simulink model "VSM_specComp_DC_22a"  (R2022a)
settings: Solver=ode3  StartTime=0.0  StopTime=4  FixedStep=HWSampleTime  RelTol=1e-3
PostLoadFcn:
  | EXEC_MODE=ExecutionMode.SIMULATION;
  | %Sim_TP33_VSM_HSS_init
InitFcn:
  | %EXEC_MODE=ExecutionMode.SIMULATION;
  | %Sim_TP33_VSM_HSS_init
StopFcn:
  | %sim2struct
undefined symbols (not defined in the file): ControlSampleTime, DiscIntNeverNeededParam, fault_dur, Grid, HWSampleTime, Ion, LCL, Lithium, Manage, Param, SM, t_fault, V_DC, VSMCTRL
libraries: FriedrichLibrary x76, simulink x32, TriphaseHardwaremodule x24, spsThreePhaseSeriesRLCBranchLib x8, spsThreePhaseVIMeasurementLib x8, spsThreePhaseBreakerLib x8, spsGroundLib x4, spsUniversalBridgeLib x4, spsVoltageMeasurementLib x4, spsEdgeDetectorLib x4, spsMeanLib x4, simulink_extras x4
(part 2 of 10)

== system VSM_specComp_DC_22a/VSM_1/VSM1/MeasInv1 ==
  SimOut : Inport
  Bus Selector1 : BusSelector  OutputSignals=meas_u_dc,meas_u_cap,meas_u_out,meas_i_inverter,meas_i_out,connection_state,enabled
  Meas_Inv1 : Scope  NumInputPorts=7
  To Workspace1 : ToWorkspace  VariableName=MeasAC_Ucap  SampleTime=-1
  To Workspace2 : ToWorkspace  VariableName=MeasAC_Uout  SampleTime=-1
  To Workspace3 : ToWorkspace  VariableName=MeasAC_Iinv  SampleTime=-1
  To Workspace4 : ToWorkspace  VariableName=MeasAC_Iout  SampleTime=-1
  To Workspace7 : ToWorkspace  VariableName=MeasAC_Udc  SampleTime=-1
  wires:
  Bus Selector1/7 -> Meas_Inv1/7  "<enabled>"
  Bus Selector1/6 -> Meas_Inv1/6  "<connection_state>"
  Bus Selector1/5 -> To Workspace4/1, Meas_Inv1/5  "<meas_i_out>"
  Bus Selector1/4 -> To Workspace3/1, Meas_Inv1/4  "<meas_i_inverter>"
  Bus Selector1/3 -> To Workspace2/1, Meas_Inv1/3  "<meas_u_out>"
  Bus Selector1/2 -> To Workspace1/1, Meas_Inv1/2  "<meas_u_cap>"
  Bus Selector1/1 -> To Workspace7/1, Meas_Inv1/1  "<meas_u_dc>"
  SimOut/1 -> Bus Selector1/1

== system VSM_specComp_DC_22a/VSM_1/VSM1/VSM ==
  cmd : Inport
  meas : Inport  Port=2
  BUS_GENERATION : Subsystem
  CONTROL : Subsystem
  MANAGEMENT : Subsystem  mask(VSMCC Management){Mgn=Ctrl.Mgn}
      mask prompts: Mgn "Mgn Parameters"
      mask help:
      | Mgn(.PQSpRateUp, .PQSpRateDown, PQSpMax, .PQSpMin)
      |
      | Parameter nicht auf der Maske:
      | ControlSampleTime
  Meas : Subsystem  mask(Messeinrichtung für VSM mit CC){PU=pu, PLL=Ctrl.PLL}
      mask prompts: PU "PU System"; PLL "PLL Parameters"
      mask help:
      | PU System(.Vb, .Ib)
      |
      | PLL Parameter (.kp, .ki)
      |
      | Parameter nicht auf der Maske:
      | NrChannels
      | ControlSampleTime
  ctrl : Outport  VectorParamsAs1DForOutWhenUnconnected=off  LockScale=on
  feedback : Outport  Port=2  VectorParamsAs1DForOutWhenUnconnected=off
  diag : Outport  Port=3  VectorParamsAs1DForOutWhenUnconnected=off
  wires:
  meas/1 -> Meas/1(MEASIN)
  cmd/1 -> MANAGEMENT/1(CMD)
  CONTROL/1(CONTROL) -> Meas/2("CONTROL "), BUS_GENERATION/2(CONTROL)
  BUS_GENERATION/1(ctrl) -> ctrl/1
  BUS_GENERATION/2(feedback) -> feedback/1
  CONTROL/2(diagCtrl) -> diag/1
  MANAGEMENT/1(MANAGE) -> CONTROL/1(MANAGE), BUS_GENERATION/1(MANAGE)
  Meas/1(MEAS) -> CONTROL/2(MEAS), MANAGEMENT/2(MEAS)

== system VSM_specComp_DC_22a/VSM_1/VSM1/command_center ==
  note: State Machine for TP <-> WP SIM
      |
      | State Index:
      | 0: Error
      | 1: Stop
      | 2: Ready (Precharge, Connected + Enable DC)
      | 3: Connect AC
      | 4: Enable AC
  Feed_AC : Inport
  Feed_DC : Inport  Port=2
  Bus Assignment : BusAssignment  AssignedSignals=Manage.connect,Manage.enable,Param.VSM.sp_PQ,Param.VSM.sp_E
  Bus Selector2 : BusSelector  OutputSignals=connect,enable
  Bus Creator1 : BusCreator  Inputs=2
  Constant2 : Constant  Value=1.01
  Display1 : Display
  Display2 : Display
  Display5 : Display
  Error ACK : Subsystem
      settings: OpenFcn=|
      | switch get_param([gcb '/Toggle'],'Value')
      |     case '1'
      |         set_param([gcb '/Toggle'],'Value', '0');
      |         set_param(gcb,'BackgroundColor','[0.8500    0.3250    0.0980]');
      |     case '0'
      |         set_param([gcb '/Toggle'],'Value', '1');
      |         set_param(gcb,'BackgroundColor','[0.4660    0.6740    0.1880]');
      | end
      mask Display: port_label('output',1,'')
  Rate Transition3 : RateTransition  Integrity=off  OutPortSampleTime=ControlSampleTime
  Shortcut1 : Subsystem  mask{path=./ControlLibrary/FriedrichLibrary.slx}
      settings: OpenFcn=findsimscopes
      mask Display: disp('Open Scopes...')
  Step3 : Step  Time=5.0+100  Before=[0.5 0]  After=[0.1 0]  SampleTime=0
  Step4 : Step  Time=0  SampleTime=0
  Subsystem : Subsystem
  cmd_VSM : Subsystem  AncestorBlock=ControLibrary/cmd_VSM template
  cmd_tp : Outport  VectorParamsAs1DForOutWhenUnconnected=off
  cmd_ac : Outport  Port=2  VectorParamsAs1DForOutWhenUnconnected=off
  wires:
  Rate Transition3/1 -> cmd_ac/1
  cmd_VSM/1(cmd_ac) -> Bus Assignment/1
  Bus Assignment/1 -> Rate Transition3/1
  Error ACK/1(Out) -> Bus Creator1/1  "error_ack"
  Bus Creator1/1 -> cmd_tp/1
  Subsystem/1(precharge) -> Bus Creator1/2, Display5/1
  Feed_AC/1 -> Subsystem/1(In1)
  Feed_DC/1 -> Subsystem/2(In2)
  Subsystem/2(cmd_ac) -> Bus Selector2/1
  Step4/1 -> Subsystem/Enable
  Step3/1 -> Bus Assignment/4
  Constant2/1 -> Bus Assignment/5
  Bus Selector2/1 -> Display1/1, Bus Assignment/2  "<connect>"
  Bus Selector2/2 -> Display2/1, Bus Assignment/3  "<enable>"

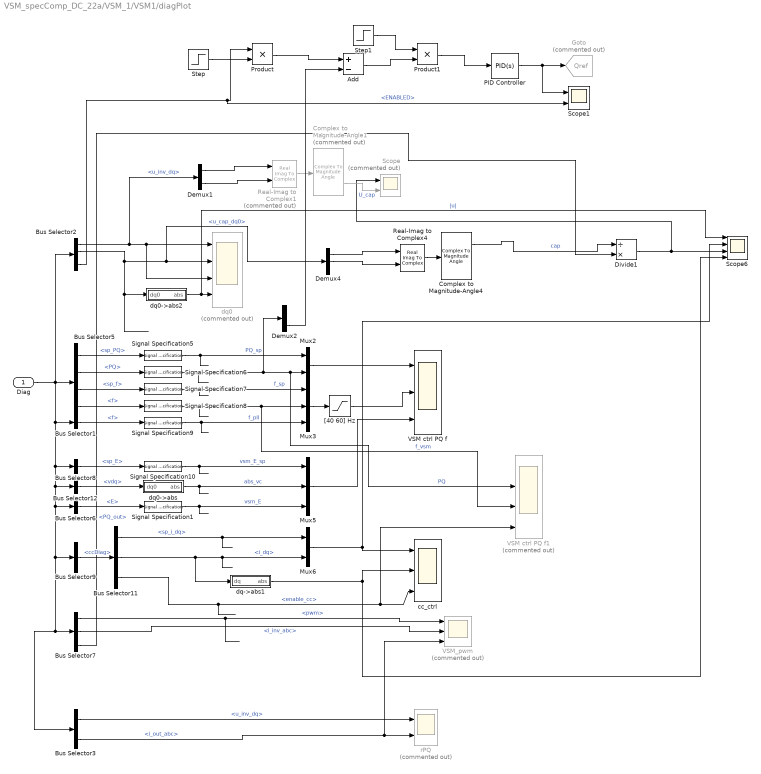
== system VSM_specComp_DC_22a/VSM_1/VSM1/diagPlot ==
  Diag : Inport
  Add : Sum  Inputs=+-
  Bus Selector1 : BusSelector  OutputSignals=measDiag.PLL.f
  Bus Selector11 : BusSelector  OutputSignals=sp_i_dq,i_dq,enable_cc
  Bus Selector12 : BusSelector  OutputSignals=measDiag.PLL.vdq
  Bus Selector2 : BusSelector  OutputSignals=u_inv_dq,measDiag.u_cap.u_cap_dq0,measDiag.u_cap.u_cap_abc,manage.ENABLED
  Bus Selector3 : BusSelector  OutputSignals=u_inv_dq,measDiag.i_out.i_out_abc
  Bus Selector5 : BusSelector  OutputSignals=manage.sp_VSM.sp_PQ,measDiag.PQ,manage.sp_VSM.sp_f,vsmDiag.f
  Bus Selector6 : BusSelector  OutputSignals=vsmDiag.E
  Bus Selector7 : BusSelector  OutputSignals=pwmDiag.pwm,measDiag.i_inv.i_inv_abc,measDiag.PQ_out
  Bus Selector8 : BusSelector  OutputSignals=vsmDiag.sp_VSM.sp_E
  Bus Selector9 : BusSelector  OutputSignals=ccDiag
  Complex to Magnitude-Angle1 : ComplexToMagnitudeAngle  Commented=on
  Complex to Magnitude-Angle4 : ComplexToMagnitudeAngle
  Demux1 : Demux  Outputs=2
  Demux2 : Demux  Outputs=2
  Demux4 : Demux  Outputs=3
  Divide1 : Product  Inputs=/*
  Goto : Goto  Commented=on  GotoTag=Qref  TagVisibility=global
  Mux2 : Mux  Inputs=2
  Mux3 : Mux  Inputs=3
  Mux5 : Mux  Inputs=3
  Mux6 : Mux  Inputs=2
  PID Controller : slpidlib/PID Controller  Controller=PID  Form=Parallel  TimeDomain=Continuous-time  UseExternalTs=off  SampleTime=-1  IntegratorMethod=Forward Euler  FilterMethod=Forward Euler  ControllerParametersSource=internal  P=0.1  I=1  UseKiTs=off  D=0  N=100  UseFilter=on  TunerSelectOption=Transfer Function Based (PID Tuner App)  InitialConditionSource=internal  InitialConditionForIntegrator=1.085  InitialConditionForFilter=0  DifferentiatorICPrevScaledInput=0  ExternalReset=none  TrackingMode=off  Kt=1  LimitOutput=off  SatLimitsSource=internal  UpperSaturationLimit=inf  LowerSaturationLimit=-inf  LinearizeAsGain=on  AntiWindupMode=none  Kb=1  POutMin=[]  POutMax=[]  IOutMin=[]  IOutMax=[]  DOutMin=[]  DOutMax=[]  NOutMin=[]  NOutMax=[]  SumOutMin=[]  SumOutMax=[]  SaturationOutMin=[]  SaturationOutMax=[]  PParamMin=[]  PParamMax=[]  IParamMin=[]  IParamMax=[]  DParamMin=[]  DParamMax=[]  NParamMin=[]  NParamMax=[]  KbParamMin=[]  KbParamMax=[]  KtParamMin=[]  KtParamMax=[]  KbOutMin=[]  KbOutMax=[]  KtOutMin=[]  KtOutMax=[]  IntegratorOutMin=[]  IntegratorOutMax=[]  FilterOutMin=[]  FilterOutMax=[]  SumI1OutMin=[]  SumI1OutMax=[]  SumI2OutMin=[]  SumI2OutMax=[]  SumI3OutMin=[]  SumI3OutMax=[]  SumI4OutMin=[]  SumI4OutMax=[]  SumDOutMin=[]  SumDOutMax=[]  DifferentiatorOutMin=[]  DifferentiatorOutMax=[]  FilterDiffOutCoefMin=[]  FilterDiffOutCoefMax=[]  ReciprocalOutMin=[]  ReciprocalOutMax=[]  SumDenOutMin=[]  SumDenOutMax=[]  SumNumOutMin=[]  SumNumOutMax=[]  DivideOutMin=[]  DivideOutMax=[]  UdiffTsProdOutMin=[]  UdiffTsProdOutMax=[]  NTsProdOutMin=[]  NTsProdOutMax=[]  UintegralTsProdOutMin=[]  UintegralTsProdOutMax=[]  UngainTsProdOutMin=[]  UngainTsProdOutMax=[]  IntegratorContinuousStateAttributes=''  IntegratorStateMustResolveToSignalObject=off  IntegratorRTWStateStorageClass=Auto  FilterContinuousStateAttributes=''  FilterStateMustResolveToSignalObject=off  FilterRTWStateStorageClass=Auto  ParallelPVariant=InternalParameters  IdealPVariant=Disabled  IVariant=InternalParameters  DVariant=InternalParameters  IntegratorVariant=Continuous  SatVariant=Disabled  AWVariant=Passthrough  PCopyVariant=Disabled  TRVariant=Disabled  FdbkBlocksVariant=Forward  IdealPFdbkVariant=Disabled  SatFdbkVariant=Disabled  DerivativeFilterVariant=ContFilter  NVariant=InternalParameters  NCopyVariant=Disabled  FilterICVariant=InternalICsFilter  IntegratorICVariant=InternalICs  ExternalResetVariant=Disabled  TRSumVariant=Passthrough  SumFdbkVariant=Disabled  SumVariant=Sum_PID  TsampFilterVariant=InternalTs  TsampNgainVariant=Passthrough  TsampIntegralVariant=Disabled_SignalSpec  ExternalSaturationOutDataTypeStr=Inherit: Same as second input
  Product : Product
  Product1 : Product
  Real-Imag to Complex1 : RealImagToComplex  Commented=on
  Real-Imag to Complex4 : RealImagToComplex
  Scope : Scope  Commented=on  NumInputPorts=2
  Scope1 : Scope  NumInputPorts=2
  Scope6 : Scope  NumInputPorts=4
  Signal Specification{1,5..10} (7 alike) : SignalSpecification
  Step : Step  Time=6+10  Before=0.1  After=0.5  SampleTime=0
  Step1 : Step  Time=6+10  SampleTime=0
  VSM ctrl PQ f : Scope  NumInputPorts=3
  VSM ctrl PQ f1 : Scope  Commented=on  NumInputPorts=4
  VSM_pwm : Scope  Commented=on  NumInputPorts=3
  "[40 60] Hz" : Saturate  UpperLimit=60  LowerLimit=40
  cc_ctrl : Scope  NumInputPorts=3
  dq->abs1 : Subsystem
  dq0 : Scope  Commented=on  NumInputPorts=4
  dq0->abs : Subsystem
  dq0->abs2 : Subsystem
  rPQ : Scope  Commented=on  NumInputPorts=2
  wires:
  Diag/1 -> Bus Selector2/1, Bus Selector6/1, Bus Selector7/1, Bus Selector3/1, Bus Selector9/1, Bus Selector12/1, Bus Selector8/1, Bus Selector1/1, Bus Selector5/1
  Bus Selector7/1 -> VSM_pwm/1  "<pwm>"
  Mux5/1 -> VSM ctrl PQ f/3
  dq0->abs/1(abs) -> Mux5/2  "abs_vc"
  Bus Selector8/1 -> Signal Specification10/1  "<sp_E>"
  Bus Selector11/1 -> Mux6/1  "<sp_i_dq>"
  Bus Selector9/1 -> Bus Selector11/1  "<ccDiag>"
  Bus Selector12/1 -> dq0->abs/1(dq0)  "<vdq>"
  Bus Selector11/3 -> VSM ctrl PQ f1/4, cc_ctrl/3  "<enable_cc>"
  Mux6/1 -> Scope6/2, cc_ctrl/1
  Bus Selector5/1 -> Signal Specification5/1  "<sp_PQ>"
  Bus Selector5/2 -> Signal Specification6/1  "<PQ>"
  Bus Selector5/3 -> Signal Specification7/1  "<sp_f>"
  Bus Selector5/4 -> Signal Specification8/1  "<f>"
  Signal Specification5/1 -> Mux2/1  "PQ_sp"
  Signal Specification7/1 -> Mux3/1  "f_sp"
  Signal Specification8/1 -> VSM ctrl PQ f1/3, Mux3/2  "f_vsm"
  Mux2/1 -> VSM ctrl PQ f/1
  Mux3/1 -> "[40 60] Hz"/1
  Bus Selector1/1 -> Signal Specification9/1  "<f>"
  Signal Specification9/1 -> Mux3/3  "f_pll"
  Signal Specification10/1 -> Mux5/1  "vsm_E_sp"
  Bus Selector11/2 -> dq->abs1/1(dq), Mux6/2  "<i_dq>"
  dq->abs1/1(abs) -> cc_ctrl/2, Scope6/4
  Bus Selector6/1 -> Signal Specification1/1  "<E>"
  Signal Specification1/1 -> Mux5/3  "vsm_E"
  "[40 60] Hz"/1 -> VSM ctrl PQ f/2
  dq0->abs2/1(abs) -> Scope6/1, dq0/4  "|u|"
  Bus Selector3/2 -> VSM_pwm/3, rPQ/2  "<i_out_abc>"
  Bus Selector3/1 -> rPQ/1  "<u_inv_dq>"
  Bus Selector7/2 -> VSM_pwm/2  "<i_inv_abc>"
  Bus Selector2/2 -> dq0->abs2/1(dq0), Demux4/1, dq0/2  "<u_cap_dq0>"
  Real-Imag to Complex4/1 -> Complex to Magnitude-Angle4/1
  Demux4/1 -> Real-Imag to Complex4/1
  Demux4/2 -> Real-Imag to Complex4/2
  Complex to Magnitude-Angle4/1 -> Divide1/1  "cap"
  Signal Specification6/1 -> Demux2/1, VSM ctrl PQ f1/2, Mux2/2  "PQ"
  Bus Selector7/3 -> Divide1/2  "<PQ_out>"
  Divide1/1 -> Scope/1, Scope6/3
  Demux1/2 -> Real-Imag to Complex1/2
  Demux1/1 -> Real-Imag to Complex1/1
  Real-Imag to Complex1/1 -> Complex to Magnitude-Angle1/1
  Complex to Magnitude-Angle1/2 -> Scope/2  "U_cap"
  Bus Selector2/1 -> Demux1/1, dq0/3, dq0/1  "<u_inv_dq>"
  Demux2/2 -> Add/2
  PID Controller/1 -> Scope1/1, Goto/1
  Step/1 -> Product/2
  Product/1 -> Add/1
  Bus Selector2/4 -> Scope1/2, Product/1  "<ENABLED>"
  Add/1 -> Product1/2
  Product1/1 -> PID Controller/1
  Step1/1 -> Product1/1

== system VSM_specComp_DC_22a/VSM_2/VSM1/MeasInv1 ==
  SimOut : Inport
  Bus Selector1 : BusSelector  OutputSignals=meas_u_dc,meas_u_cap,meas_u_out,meas_i_inverter,meas_i_out,connection_state,enabled
  Meas_Inv1 : Scope  NumInputPorts=7
  To Workspace1 : ToWorkspace  VariableName=MeasAC_Ucap  SampleTime=-1
  To Workspace2 : ToWorkspace  VariableName=MeasAC_Uout  SampleTime=-1
  To Workspace3 : ToWorkspace  VariableName=MeasAC_Iinv  SampleTime=-1
  To Workspace4 : ToWorkspace  VariableName=MeasAC_Iout  SampleTime=-1
  To Workspace7 : ToWorkspace  VariableName=MeasAC_Udc  SampleTime=-1
  wires:
  Bus Selector1/7 -> Meas_Inv1/7  "<enabled>"
  Bus Selector1/6 -> Meas_Inv1/6  "<connection_state>"
  Bus Selector1/5 -> To Workspace4/1, Meas_Inv1/5  "<meas_i_out>"
  Bus Selector1/4 -> To Workspace3/1, Meas_Inv1/4  "<meas_i_inverter>"
  Bus Selector1/3 -> To Workspace2/1, Meas_Inv1/3  "<meas_u_out>"
  Bus Selector1/2 -> To Workspace1/1, Meas_Inv1/2  "<meas_u_cap>"
  Bus Selector1/1 -> To Workspace7/1, Meas_Inv1/1  "<meas_u_dc>"
  SimOut/1 -> Bus Selector1/1

== system VSM_specComp_DC_22a/VSM_2/VSM1/VSM ==
  cmd : Inport
  meas : Inport  Port=2
  BUS_GENERATION : Subsystem
  CONTROL : Subsystem
  MANAGEMENT : Subsystem  mask(VSMCC Management){Mgn=Ctrl.Mgn}
      mask prompts: Mgn "Mgn Parameters"
      mask help:
      | Mgn(.PQSpRateUp, .PQSpRateDown, PQSpMax, .PQSpMin)
      |
      | Parameter nicht auf der Maske:
      | ControlSampleTime
  Meas : Subsystem  mask(Messeinrichtung für VSM mit CC){PU=pu, PLL=Ctrl.PLL}
      mask prompts: PU "PU System"; PLL "PLL Parameters"
      mask help:
      | PU System(.Vb, .Ib)
      |
      | PLL Parameter (.kp, .ki)
      |
      | Parameter nicht auf der Maske:
      | NrChannels
      | ControlSampleTime
  ctrl : Outport  VectorParamsAs1DForOutWhenUnconnected=off  LockScale=on
  feedback : Outport  Port=2  VectorParamsAs1DForOutWhenUnconnected=off
  diag : Outport  Port=3  VectorParamsAs1DForOutWhenUnconnected=off
  wires:
  meas/1 -> Meas/1(MEASIN)
  cmd/1 -> MANAGEMENT/1(CMD)
  CONTROL/1(CONTROL) -> Meas/2("CONTROL "), BUS_GENERATION/2(CONTROL)
  BUS_GENERATION/1(ctrl) -> ctrl/1
  BUS_GENERATION/2(feedback) -> feedback/1
  CONTROL/2(diagCtrl) -> diag/1
  MANAGEMENT/1(MANAGE) -> CONTROL/1(MANAGE), BUS_GENERATION/1(MANAGE)
  Meas/1(MEAS) -> CONTROL/2(MEAS), MANAGEMENT/2(MEAS)

== system VSM_specComp_DC_22a/VSM_2/VSM1/command_center ==
  note: State Machine for TP <-> WP SIM
      |
      | State Index:
      | 0: Error
      | 1: Stop
      | 2: Ready (Precharge, Connected + Enable DC)
      | 3: Connect AC
      | 4: Enable AC
  Feed_AC : Inport
  Feed_DC : Inport  Port=2
  Bus Assignment : BusAssignment  AssignedSignals=Manage.connect,Manage.enable,Param.VSM.sp_PQ,Param.VSM.sp_E
  Bus Selector2 : BusSelector  OutputSignals=connect,enable
  Bus Creator1 : BusCreator  Inputs=2
  Constant2 : Constant  Value=1.01
  Display1 : Display
  Display2 : Display
  Display5 : Display
  Error ACK : Subsystem
      settings: OpenFcn=|
      | switch get_param([gcb '/Toggle'],'Value')
      |     case '1'
      |         set_param([gcb '/Toggle'],'Value', '0');
      |         set_param(gcb,'BackgroundColor','[0.8500    0.3250    0.0980]');
      |     case '0'
      |         set_param([gcb '/Toggle'],'Value', '1');
      |         set_param(gcb,'BackgroundColor','[0.4660    0.6740    0.1880]');
      | end
      mask Display: port_label('output',1,'')
  Rate Transition3 : RateTransition  Integrity=off  OutPortSampleTime=ControlSampleTime
  Shortcut1 : Subsystem  mask{path=./ControlLibrary/FriedrichLibrary.slx}
      settings: OpenFcn=findsimscopes
      mask Display: disp('Open Scopes...')
  Step3 : Step  Time=5.0+100  Before=[0.5 0]  After=[0.1 0]  SampleTime=0
  Step4 : Step  Time=0  SampleTime=0
  Subsystem : Subsystem
  cmd_VSM : Subsystem  AncestorBlock=ControLibrary/cmd_VSM template
  cmd_tp : Outport  VectorParamsAs1DForOutWhenUnconnected=off
  cmd_ac : Outport  Port=2  VectorParamsAs1DForOutWhenUnconnected=off
  wires:
  Rate Transition3/1 -> cmd_ac/1
  cmd_VSM/1(cmd_ac) -> Bus Assignment/1
  Bus Assignment/1 -> Rate Transition3/1
  Error ACK/1(Out) -> Bus Creator1/1  "error_ack"
  Bus Creator1/1 -> cmd_tp/1
  Subsystem/1(precharge) -> Bus Creator1/2, Display5/1
  Feed_AC/1 -> Subsystem/1(In1)
  Feed_DC/1 -> Subsystem/2(In2)
  Subsystem/2(cmd_ac) -> Bus Selector2/1
  Step4/1 -> Subsystem/Enable
  Step3/1 -> Bus Assignment/4
  Constant2/1 -> Bus Assignment/5
  Bus Selector2/1 -> Display1/1, Bus Assignment/2  "<connect>"
  Bus Selector2/2 -> Display2/1, Bus Assignment/3  "<enable>"

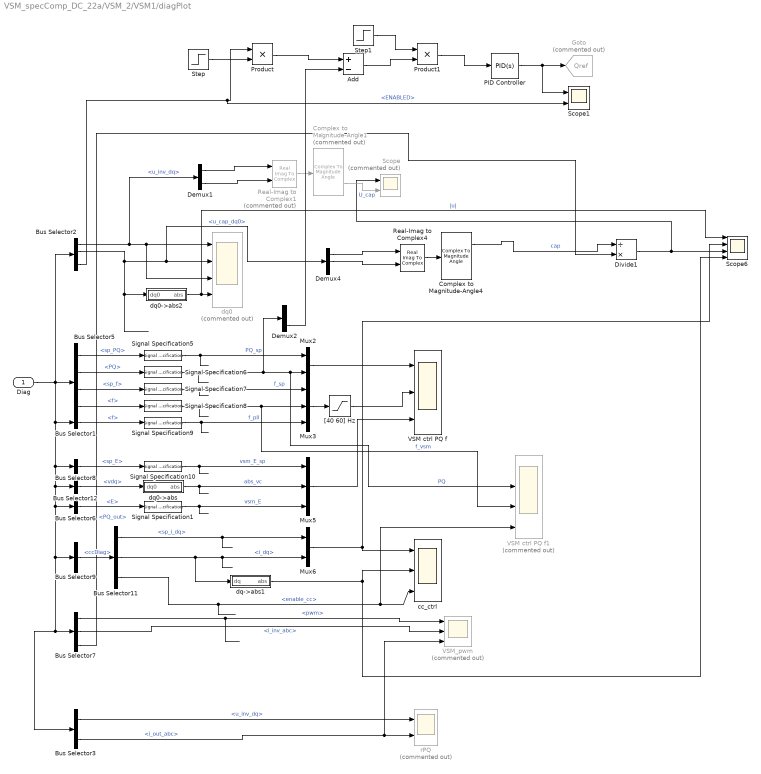
== system VSM_specComp_DC_22a/VSM_2/VSM1/diagPlot ==
  Diag : Inport
  Add : Sum  Inputs=+-
  Bus Selector1 : BusSelector  OutputSignals=measDiag.PLL.f
  Bus Selector11 : BusSelector  OutputSignals=sp_i_dq,i_dq,enable_cc
  Bus Selector12 : BusSelector  OutputSignals=measDiag.PLL.vdq
  Bus Selector2 : BusSelector  OutputSignals=u_inv_dq,measDiag.u_cap.u_cap_dq0,measDiag.u_cap.u_cap_abc,manage.ENABLED
  Bus Selector3 : BusSelector  OutputSignals=u_inv_dq,measDiag.i_out.i_out_abc
  Bus Selector5 : BusSelector  OutputSignals=manage.sp_VSM.sp_PQ,measDiag.PQ,manage.sp_VSM.sp_f,vsmDiag.f
  Bus Selector6 : BusSelector  OutputSignals=vsmDiag.E
  Bus Selector7 : BusSelector  OutputSignals=pwmDiag.pwm,measDiag.i_inv.i_inv_abc,measDiag.PQ_out
  Bus Selector8 : BusSelector  OutputSignals=vsmDiag.sp_VSM.sp_E
  Bus Selector9 : BusSelector  OutputSignals=ccDiag
  Complex to Magnitude-Angle1 : ComplexToMagnitudeAngle  Commented=on
  Complex to Magnitude-Angle4 : ComplexToMagnitudeAngle
  Demux1 : Demux  Outputs=2
  Demux2 : Demux  Outputs=2
  Demux4 : Demux  Outputs=3
  Divide1 : Product  Inputs=/*
  Goto : Goto  Commented=on  GotoTag=Qref  TagVisibility=global
  Mux2 : Mux  Inputs=2
  Mux3 : Mux  Inputs=3
  Mux5 : Mux  Inputs=3
  Mux6 : Mux  Inputs=2
  PID Controller : slpidlib/PID Controller  Controller=PID  Form=Parallel  TimeDomain=Continuous-time  UseExternalTs=off  SampleTime=-1  IntegratorMethod=Forward Euler  FilterMethod=Forward Euler  ControllerParametersSource=internal  P=0.1  I=1  UseKiTs=off  D=0  N=100  UseFilter=on  TunerSelectOption=Transfer Function Based (PID Tuner App)  InitialConditionSource=internal  InitialConditionForIntegrator=1.085  InitialConditionForFilter=0  DifferentiatorICPrevScaledInput=0  ExternalReset=none  TrackingMode=off  Kt=1  LimitOutput=off  SatLimitsSource=internal  UpperSaturationLimit=inf  LowerSaturationLimit=-inf  LinearizeAsGain=on  AntiWindupMode=none  Kb=1  POutMin=[]  POutMax=[]  IOutMin=[]  IOutMax=[]  DOutMin=[]  DOutMax=[]  NOutMin=[]  NOutMax=[]  SumOutMin=[]  SumOutMax=[]  SaturationOutMin=[]  SaturationOutMax=[]  PParamMin=[]  PParamMax=[]  IParamMin=[]  IParamMax=[]  DParamMin=[]  DParamMax=[]  NParamMin=[]  NParamMax=[]  KbParamMin=[]  KbParamMax=[]  KtParamMin=[]  KtParamMax=[]  KbOutMin=[]  KbOutMax=[]  KtOutMin=[]  KtOutMax=[]  IntegratorOutMin=[]  IntegratorOutMax=[]  FilterOutMin=[]  FilterOutMax=[]  SumI1OutMin=[]  SumI1OutMax=[]  SumI2OutMin=[]  SumI2OutMax=[]  SumI3OutMin=[]  SumI3OutMax=[]  SumI4OutMin=[]  SumI4OutMax=[]  SumDOutMin=[]  SumDOutMax=[]  DifferentiatorOutMin=[]  DifferentiatorOutMax=[]  FilterDiffOutCoefMin=[]  FilterDiffOutCoefMax=[]  ReciprocalOutMin=[]  ReciprocalOutMax=[]  SumDenOutMin=[]  SumDenOutMax=[]  SumNumOutMin=[]  SumNumOutMax=[]  DivideOutMin=[]  DivideOutMax=[]  UdiffTsProdOutMin=[]  UdiffTsProdOutMax=[]  NTsProdOutMin=[]  NTsProdOutMax=[]  UintegralTsProdOutMin=[]  UintegralTsProdOutMax=[]  UngainTsProdOutMin=[]  UngainTsProdOutMax=[]  IntegratorContinuousStateAttributes=''  IntegratorStateMustResolveToSignalObject=off  IntegratorRTWStateStorageClass=Auto  FilterContinuousStateAttributes=''  FilterStateMustResolveToSignalObject=off  FilterRTWStateStorageClass=Auto  ParallelPVariant=InternalParameters  IdealPVariant=Disabled  IVariant=InternalParameters  DVariant=InternalParameters  IntegratorVariant=Continuous  SatVariant=Disabled  AWVariant=Passthrough  PCopyVariant=Disabled  TRVariant=Disabled  FdbkBlocksVariant=Forward  IdealPFdbkVariant=Disabled  SatFdbkVariant=Disabled  DerivativeFilterVariant=ContFilter  NVariant=InternalParameters  NCopyVariant=Disabled  FilterICVariant=InternalICsFilter  IntegratorICVariant=InternalICs  ExternalResetVariant=Disabled  TRSumVariant=Passthrough  SumFdbkVariant=Disabled  SumVariant=Sum_PID  TsampFilterVariant=InternalTs  TsampNgainVariant=Passthrough  TsampIntegralVariant=Disabled_SignalSpec  ExternalSaturationOutDataTypeStr=Inherit: Same as second input
  Product : Product
  Product1 : Product
  Real-Imag to Complex1 : RealImagToComplex  Commented=on
  Real-Imag to Complex4 : RealImagToComplex
  Scope : Scope  Commented=on  NumInputPorts=2
  Scope1 : Scope  NumInputPorts=2
  Scope6 : Scope  NumInputPorts=4
  Signal Specification{1,5..10} (7 alike) : SignalSpecification
  Step : Step  Time=6+10  Before=0.1  After=0.5  SampleTime=0
  Step1 : Step  Time=6+10  SampleTime=0
  VSM ctrl PQ f : Scope  NumInputPorts=3
  VSM ctrl PQ f1 : Scope  Commented=on  NumInputPorts=4
  VSM_pwm : Scope  Commented=on  NumInputPorts=3
  "[40 60] Hz" : Saturate  UpperLimit=60  LowerLimit=40
  cc_ctrl : Scope  NumInputPorts=3
  dq->abs1 : Subsystem
  dq0 : Scope  Commented=on  NumInputPorts=4
  dq0->abs : Subsystem
  dq0->abs2 : Subsystem
  rPQ : Scope  Commented=on  NumInputPorts=2
  wires:
  Diag/1 -> Bus Selector2/1, Bus Selector6/1, Bus Selector7/1, Bus Selector3/1, Bus Selector9/1, Bus Selector12/1, Bus Selector8/1, Bus Selector1/1, Bus Selector5/1
  Bus Selector7/1 -> VSM_pwm/1  "<pwm>"
  Mux5/1 -> VSM ctrl PQ f/3
  dq0->abs/1(abs) -> Mux5/2  "abs_vc"
  Bus Selector8/1 -> Signal Specification10/1  "<sp_E>"
  Bus Selector11/1 -> Mux6/1  "<sp_i_dq>"
  Bus Selector9/1 -> Bus Selector11/1  "<ccDiag>"
  Bus Selector12/1 -> dq0->abs/1(dq0)  "<vdq>"
  Bus Selector11/3 -> VSM ctrl PQ f1/4, cc_ctrl/3  "<enable_cc>"
  Mux6/1 -> Scope6/2, cc_ctrl/1
  Bus Selector5/1 -> Signal Specification5/1  "<sp_PQ>"
  Bus Selector5/2 -> Signal Specification6/1  "<PQ>"
  Bus Selector5/3 -> Signal Specification7/1  "<sp_f>"
  Bus Selector5/4 -> Signal Specification8/1  "<f>"
  Signal Specification5/1 -> Mux2/1  "PQ_sp"
  Signal Specification7/1 -> Mux3/1  "f_sp"
  Signal Specification8/1 -> VSM ctrl PQ f1/3, Mux3/2  "f_vsm"
  Mux2/1 -> VSM ctrl PQ f/1
  Mux3/1 -> "[40 60] Hz"/1
  Bus Selector1/1 -> Signal Specification9/1  "<f>"
  Signal Specification9/1 -> Mux3/3  "f_pll"
  Signal Specification10/1 -> Mux5/1  "vsm_E_sp"
  Bus Selector11/2 -> dq->abs1/1(dq), Mux6/2  "<i_dq>"
  dq->abs1/1(abs) -> cc_ctrl/2, Scope6/4
  Bus Selector6/1 -> Signal Specification1/1  "<E>"
  Signal Specification1/1 -> Mux5/3  "vsm_E"
  "[40 60] Hz"/1 -> VSM ctrl PQ f/2
  dq0->abs2/1(abs) -> Scope6/1, dq0/4  "|u|"
  Bus Selector3/2 -> VSM_pwm/3, rPQ/2  "<i_out_abc>"
  Bus Selector3/1 -> rPQ/1  "<u_inv_dq>"
  Bus Selector7/2 -> VSM_pwm/2  "<i_inv_abc>"
  Bus Selector2/2 -> dq0->abs2/1(dq0), Demux4/1, dq0/2  "<u_cap_dq0>"
  Real-Imag to Complex4/1 -> Complex to Magnitude-Angle4/1
  Demux4/1 -> Real-Imag to Complex4/1
  Demux4/2 -> Real-Imag to Complex4/2
  Complex to Magnitude-Angle4/1 -> Divide1/1  "cap"
  Signal Specification6/1 -> Demux2/1, VSM ctrl PQ f1/2, Mux2/2  "PQ"
  Bus Selector7/3 -> Divide1/2  "<PQ_out>"
  Divide1/1 -> Scope/1, Scope6/3
  Demux1/2 -> Real-Imag to Complex1/2
  Demux1/1 -> Real-Imag to Complex1/1
  Real-Imag to Complex1/1 -> Complex to Magnitude-Angle1/1
  Complex to Magnitude-Angle1/2 -> Scope/2  "U_cap"
  Bus Selector2/1 -> Demux1/1, dq0/3, dq0/1  "<u_inv_dq>"
  Demux2/2 -> Add/2
  PID Controller/1 -> Scope1/1, Goto/1
  Step/1 -> Product/2
  Product/1 -> Add/1
  Bus Selector2/4 -> Scope1/2, Product/1  "<ENABLED>"
  Add/1 -> Product1/2
  Product1/1 -> PID Controller/1
  Step1/1 -> Product1/1

== system VSM_specComp_DC_22a/VSM_3/VSM1/MeasInv1 ==
  SimOut : Inport
  Bus Selector1 : BusSelector  OutputSignals=meas_u_dc,meas_u_cap,meas_u_out,meas_i_inverter,meas_i_out,connection_state,enabled
  Meas_Inv1 : Scope  NumInputPorts=7
  To Workspace1 : ToWorkspace  VariableName=MeasAC_Ucap  SampleTime=-1
  To Workspace2 : ToWorkspace  VariableName=MeasAC_Uout  SampleTime=-1
  To Workspace3 : ToWorkspace  VariableName=MeasAC_Iinv  SampleTime=-1
  To Workspace4 : ToWorkspace  VariableName=MeasAC_Iout  SampleTime=-1
  To Workspace7 : ToWorkspace  VariableName=MeasAC_Udc  SampleTime=-1
  wires:
  SimOut/1 -> Bus Selector1/1
  Bus Selector1/1 -> Meas_Inv1/1, To Workspace7/1  "<meas_u_dc>"
  Bus Selector1/2 -> Meas_Inv1/2, To Workspace1/1  "<meas_u_cap>"
  Bus Selector1/3 -> Meas_Inv1/3, To Workspace2/1  "<meas_u_out>"
  Bus Selector1/4 -> Meas_Inv1/4, To Workspace3/1  "<meas_i_inverter>"
  Bus Selector1/5 -> Meas_Inv1/5, To Workspace4/1  "<meas_i_out>"
  Bus Selector1/6 -> Meas_Inv1/6  "<connection_state>"
  Bus Selector1/7 -> Meas_Inv1/7  "<enabled>"

== system VSM_specComp_DC_22a/VSM_3/VSM1/VSM ==
  cmd : Inport
  meas : Inport  Port=2
  BUS_GENERATION : Subsystem
  CONTROL : Subsystem
  MANAGEMENT : Subsystem  mask(VSMCC Management){Mgn=Ctrl.Mgn}
      mask prompts: Mgn "Mgn Parameters"
      mask help:
      | Mgn(.PQSpRateUp, .PQSpRateDown, PQSpMax, .PQSpMin)
      |
      | Parameter nicht auf der Maske:
      | ControlSampleTime
  Meas : Subsystem  mask(Messeinrichtung für VSM mit CC){PU=pu, PLL=Ctrl.PLL}
      mask prompts: PU "PU System"; PLL "PLL Parameters"
      mask help:
      | PU System(.Vb, .Ib)
      |
      | PLL Parameter (.kp, .ki)
      |
      | Parameter nicht auf der Maske:
      | NrChannels
      | ControlSampleTime
  ctrl : Outport  VectorParamsAs1DForOutWhenUnconnected=off  LockScale=on
  feedback : Outport  Port=2  VectorParamsAs1DForOutWhenUnconnected=off
  diag : Outport  Port=3  VectorParamsAs1DForOutWhenUnconnected=off
  wires:
  Meas/1(MEAS) -> MANAGEMENT/2(MEAS), CONTROL/2(MEAS)
  MANAGEMENT/1(MANAGE) -> BUS_GENERATION/1(MANAGE), CONTROL/1(MANAGE)
  CONTROL/2(diagCtrl) -> diag/1
  BUS_GENERATION/2(feedback) -> feedback/1
  BUS_GENERATION/1(ctrl) -> ctrl/1
  CONTROL/1(CONTROL) -> BUS_GENERATION/2(CONTROL), Meas/2("CONTROL ")
  cmd/1 -> MANAGEMENT/1(CMD)
  meas/1 -> Meas/1(MEASIN)

== system VSM_specComp_DC_22a/VSM_3/VSM1/command_center ==
  note: State Machine for TP <-> WP SIM
      |
      | State Index:
      | 0: Error
      | 1: Stop
      | 2: Ready (Precharge, Connected + Enable DC)
      | 3: Connect AC
      | 4: Enable AC
  Feed_AC : Inport
  Feed_DC : Inport  Port=2
  Bus Assignment : BusAssignment  AssignedSignals=Manage.connect,Manage.enable,Param.VSM.sp_PQ,Param.VSM.sp_E
  Bus Selector2 : BusSelector  OutputSignals=connect,enable
  Bus Creator1 : BusCreator  Inputs=2
  Constant2 : Constant  Value=1.01
  Display1 : Display
  Display2 : Display
  Display5 : Display
  Error ACK : Subsystem
      settings: OpenFcn=|
      | switch get_param([gcb '/Toggle'],'Value')
      |     case '1'
      |         set_param([gcb '/Toggle'],'Value', '0');
      |         set_param(gcb,'BackgroundColor','[0.8500    0.3250    0.0980]');
      |     case '0'
      |         set_param([gcb '/Toggle'],'Value', '1');
      |         set_param(gcb,'BackgroundColor','[0.4660    0.6740    0.1880]');
      | end
      mask Display: port_label('output',1,'')
  Rate Transition3 : RateTransition  Integrity=off  OutPortSampleTime=ControlSampleTime
  Shortcut1 : Subsystem  mask{path=./ControlLibrary/FriedrichLibrary.slx}
      settings: OpenFcn=findsimscopes
      mask Display: disp('Open Scopes...')
  Step3 : Step  Time=5.0+100  Before=[-0.5 0]  After=[0.1 0]  SampleTime=0
  Step4 : Step  Time=0  SampleTime=0
  Subsystem : Subsystem
  cmd_VSM : Subsystem  AncestorBlock=ControLibrary/cmd_VSM template
  cmd_tp : Outport  VectorParamsAs1DForOutWhenUnconnected=off
  cmd_ac : Outport  Port=2  VectorParamsAs1DForOutWhenUnconnected=off
  wires:
  Bus Selector2/2 -> Bus Assignment/3, Display2/1  "<enable>"
  Bus Selector2/1 -> Bus Assignment/2, Display1/1  "<connect>"
  Constant2/1 -> Bus Assignment/5
  Step3/1 -> Bus Assignment/4
  Step4/1 -> Subsystem/Enable
  Subsystem/2(cmd_ac) -> Bus Selector2/1
  Feed_DC/1 -> Subsystem/2(In2)
  Feed_AC/1 -> Subsystem/1(In1)
  Subsystem/1(precharge) -> Display5/1, Bus Creator1/2
  Bus Creator1/1 -> cmd_tp/1
  Error ACK/1(Out) -> Bus Creator1/1  "error_ack"
  Bus Assignment/1 -> Rate Transition3/1
  cmd_VSM/1(cmd_ac) -> Bus Assignment/1
  Rate Transition3/1 -> cmd_ac/1

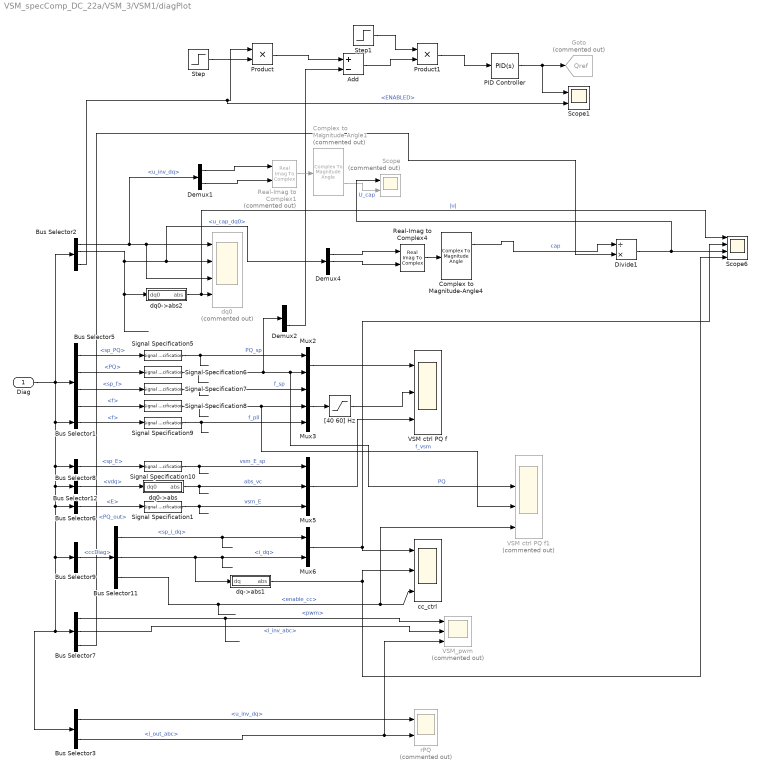
== system VSM_specComp_DC_22a/VSM_3/VSM1/diagPlot ==
  Diag : Inport
  Add : Sum  Inputs=+-
  Bus Selector1 : BusSelector  OutputSignals=measDiag.PLL.f
  Bus Selector11 : BusSelector  OutputSignals=sp_i_dq,i_dq,enable_cc
  Bus Selector12 : BusSelector  OutputSignals=measDiag.PLL.vdq
  Bus Selector2 : BusSelector  OutputSignals=u_inv_dq,measDiag.u_cap.u_cap_dq0,measDiag.u_cap.u_cap_abc,manage.ENABLED
  Bus Selector3 : BusSelector  OutputSignals=u_inv_dq,measDiag.i_out.i_out_abc
  Bus Selector5 : BusSelector  OutputSignals=manage.sp_VSM.sp_PQ,measDiag.PQ,manage.sp_VSM.sp_f,vsmDiag.f
  Bus Selector6 : BusSelector  OutputSignals=vsmDiag.E
  Bus Selector7 : BusSelector  OutputSignals=pwmDiag.pwm,measDiag.i_inv.i_inv_abc,measDiag.PQ_out
  Bus Selector8 : BusSelector  OutputSignals=vsmDiag.sp_VSM.sp_E
  Bus Selector9 : BusSelector  OutputSignals=ccDiag
  Complex to Magnitude-Angle1 : ComplexToMagnitudeAngle  Commented=on
  Complex to Magnitude-Angle4 : ComplexToMagnitudeAngle
  Demux1 : Demux  Outputs=2
  Demux2 : Demux  Outputs=2
  Demux4 : Demux  Outputs=3
  Divide1 : Product  Inputs=/*
  Goto : Goto  Commented=on  GotoTag=Qref  TagVisibility=global
  Mux2 : Mux  Inputs=2
  Mux3 : Mux  Inputs=3
  Mux5 : Mux  Inputs=3
  Mux6 : Mux  Inputs=2
  PID Controller : slpidlib/PID Controller  Controller=PID  Form=Parallel  TimeDomain=Continuous-time  UseExternalTs=off  SampleTime=-1  IntegratorMethod=Forward Euler  FilterMethod=Forward Euler  ControllerParametersSource=internal  P=0.1  I=1  UseKiTs=off  D=0  N=100  UseFilter=on  TunerSelectOption=Transfer Function Based (PID Tuner App)  InitialConditionSource=internal  InitialConditionForIntegrator=1.085  InitialConditionForFilter=0  DifferentiatorICPrevScaledInput=0  ExternalReset=none  TrackingMode=off  Kt=1  LimitOutput=off  SatLimitsSource=internal  UpperSaturationLimit=inf  LowerSaturationLimit=-inf  LinearizeAsGain=on  AntiWindupMode=none  Kb=1  POutMin=[]  POutMax=[]  IOutMin=[]  IOutMax=[]  DOutMin=[]  DOutMax=[]  NOutMin=[]  NOutMax=[]  SumOutMin=[]  SumOutMax=[]  SaturationOutMin=[]  SaturationOutMax=[]  PParamMin=[]  PParamMax=[]  IParamMin=[]  IParamMax=[]  DParamMin=[]  DParamMax=[]  NParamMin=[]  NParamMax=[]  KbParamMin=[]  KbParamMax=[]  KtParamMin=[]  KtParamMax=[]  KbOutMin=[]  KbOutMax=[]  KtOutMin=[]  KtOutMax=[]  IntegratorOutMin=[]  IntegratorOutMax=[]  FilterOutMin=[]  FilterOutMax=[]  SumI1OutMin=[]  SumI1OutMax=[]  SumI2OutMin=[]  SumI2OutMax=[]  SumI3OutMin=[]  SumI3OutMax=[]  SumI4OutMin=[]  SumI4OutMax=[]  SumDOutMin=[]  SumDOutMax=[]  DifferentiatorOutMin=[]  DifferentiatorOutMax=[]  FilterDiffOutCoefMin=[]  FilterDiffOutCoefMax=[]  ReciprocalOutMin=[]  ReciprocalOutMax=[]  SumDenOutMin=[]  SumDenOutMax=[]  SumNumOutMin=[]  SumNumOutMax=[]  DivideOutMin=[]  DivideOutMax=[]  UdiffTsProdOutMin=[]  UdiffTsProdOutMax=[]  NTsProdOutMin=[]  NTsProdOutMax=[]  UintegralTsProdOutMin=[]  UintegralTsProdOutMax=[]  UngainTsProdOutMin=[]  UngainTsProdOutMax=[]  IntegratorContinuousStateAttributes=''  IntegratorStateMustResolveToSignalObject=off  IntegratorRTWStateStorageClass=Auto  FilterContinuousStateAttributes=''  FilterStateMustResolveToSignalObject=off  FilterRTWStateStorageClass=Auto  ParallelPVariant=InternalParameters  IdealPVariant=Disabled  IVariant=InternalParameters  DVariant=InternalParameters  IntegratorVariant=Continuous  SatVariant=Disabled  AWVariant=Passthrough  PCopyVariant=Disabled  TRVariant=Disabled  FdbkBlocksVariant=Forward  IdealPFdbkVariant=Disabled  SatFdbkVariant=Disabled  DerivativeFilterVariant=ContFilter  NVariant=InternalParameters  NCopyVariant=Disabled  FilterICVariant=InternalICsFilter  IntegratorICVariant=InternalICs  ExternalResetVariant=Disabled  TRSumVariant=Passthrough  SumFdbkVariant=Disabled  SumVariant=Sum_PID  TsampFilterVariant=InternalTs  TsampNgainVariant=Passthrough  TsampIntegralVariant=Disabled_SignalSpec  ExternalSaturationOutDataTypeStr=Inherit: Same as second input
  Product : Product
  Product1 : Product
  Real-Imag to Complex1 : RealImagToComplex  Commented=on
  Real-Imag to Complex4 : RealImagToComplex
  Scope : Scope  Commented=on  NumInputPorts=2
  Scope1 : Scope  NumInputPorts=2
  Scope6 : Scope  NumInputPorts=4
  Signal Specification{1,5..10} (7 alike) : SignalSpecification
  Step : Step  Time=6+10  Before=0.1  After=0.5  SampleTime=0
  Step1 : Step  Time=6+10  SampleTime=0
  VSM ctrl PQ f : Scope  NumInputPorts=3
  VSM ctrl PQ f1 : Scope  Commented=on  NumInputPorts=4
  VSM_pwm : Scope  Commented=on  NumInputPorts=3
  "[40 60] Hz" : Saturate  UpperLimit=60  LowerLimit=40
  cc_ctrl : Scope  NumInputPorts=3
  dq->abs1 : Subsystem
  dq0 : Scope  Commented=on  NumInputPorts=4
  dq0->abs : Subsystem
  dq0->abs2 : Subsystem
  rPQ : Scope  Commented=on  NumInputPorts=2
  wires:
  Step1/1 -> Product1/1
  Product1/1 -> PID Controller/1
  Add/1 -> Product1/2
  Bus Selector2/4 -> Product/1, Scope1/2  "<ENABLED>"
  Product/1 -> Add/1
  Step/1 -> Product/2
  PID Controller/1 -> Goto/1, Scope1/1
  Demux2/2 -> Add/2
  Bus Selector2/1 -> dq0/1, dq0/3, Demux1/1  "<u_inv_dq>"
  Complex to Magnitude-Angle1/2 -> Scope/2  "U_cap"
  Real-Imag to Complex1/1 -> Complex to Magnitude-Angle1/1
  Demux1/1 -> Real-Imag to Complex1/1
  Demux1/2 -> Real-Imag to Complex1/2
  Divide1/1 -> Scope6/3, Scope/1
  Bus Selector7/3 -> Divide1/2  "<PQ_out>"
  Signal Specification6/1 -> Mux2/2, VSM ctrl PQ f1/2, Demux2/1  "PQ"
  Complex to Magnitude-Angle4/1 -> Divide1/1  "cap"
  Demux4/2 -> Real-Imag to Complex4/2
  Demux4/1 -> Real-Imag to Complex4/1
  Real-Imag to Complex4/1 -> Complex to Magnitude-Angle4/1
  Bus Selector2/2 -> dq0/2, Demux4/1, dq0->abs2/1(dq0)  "<u_cap_dq0>"
  Bus Selector7/2 -> VSM_pwm/2  "<i_inv_abc>"
  Bus Selector3/1 -> rPQ/1  "<u_inv_dq>"
  Bus Selector3/2 -> rPQ/2, VSM_pwm/3  "<i_out_abc>"
  dq0->abs2/1(abs) -> dq0/4, Scope6/1  "|u|"
  "[40 60] Hz"/1 -> VSM ctrl PQ f/2
  Signal Specification1/1 -> Mux5/3  "vsm_E"
  Bus Selector6/1 -> Signal Specification1/1  "<E>"
  dq->abs1/1(abs) -> Scope6/4, cc_ctrl/2
  Bus Selector11/2 -> Mux6/2, dq->abs1/1(dq)  "<i_dq>"
  Signal Specification10/1 -> Mux5/1  "vsm_E_sp"
  Signal Specification9/1 -> Mux3/3  "f_pll"
  Bus Selector1/1 -> Signal Specification9/1  "<f>"
  Mux3/1 -> "[40 60] Hz"/1
  Mux2/1 -> VSM ctrl PQ f/1
  Signal Specification8/1 -> Mux3/2, VSM ctrl PQ f1/3  "f_vsm"
  Signal Specification7/1 -> Mux3/1  "f_sp"
  Signal Specification5/1 -> Mux2/1  "PQ_sp"
  Bus Selector5/4 -> Signal Specification8/1  "<f>"
  Bus Selector5/3 -> Signal Specification7/1  "<sp_f>"
  Bus Selector5/2 -> Signal Specification6/1  "<PQ>"
  Bus Selector5/1 -> Signal Specification5/1  "<sp_PQ>"
  Mux6/1 -> cc_ctrl/1, Scope6/2
  Bus Selector11/3 -> cc_ctrl/3, VSM ctrl PQ f1/4  "<enable_cc>"
  Bus Selector12/1 -> dq0->abs/1(dq0)  "<vdq>"
  Bus Selector9/1 -> Bus Selector11/1  "<ccDiag>"
  Bus Selector11/1 -> Mux6/1  "<sp_i_dq>"
  Bus Selector8/1 -> Signal Specification10/1  "<sp_E>"
  dq0->abs/1(abs) -> Mux5/2  "abs_vc"
  Mux5/1 -> VSM ctrl PQ f/3
  Bus Selector7/1 -> VSM_pwm/1  "<pwm>"
  Diag/1 -> Bus Selector5/1, Bus Selector1/1, Bus Selector8/1, Bus Selector12/1, Bus Selector9/1, Bus Selector3/1, Bus Selector7/1, Bus Selector6/1, Bus Selector2/1

== system VSM_specComp_DC_22a/VSM_4/VSM1/MeasInv1 ==
  SimOut : Inport
  Bus Selector1 : BusSelector  OutputSignals=meas_u_dc,meas_u_cap,meas_u_out,meas_i_inverter,meas_i_out,connection_state,enabled
  Meas_Inv1 : Scope  NumInputPorts=7
  To Workspace1 : ToWorkspace  VariableName=MeasAC_Ucap  SampleTime=-1
  To Workspace2 : ToWorkspace  VariableName=MeasAC_Uout  SampleTime=-1
  To Workspace3 : ToWorkspace  VariableName=MeasAC_Iinv  SampleTime=-1
  To Workspace4 : ToWorkspace  VariableName=MeasAC_Iout  SampleTime=-1
  To Workspace7 : ToWorkspace  VariableName=MeasAC_Udc  SampleTime=-1
  wires:
  Bus Selector1/7 -> Meas_Inv1/7  "<enabled>"
  Bus Selector1/6 -> Meas_Inv1/6  "<connection_state>"
  Bus Selector1/5 -> To Workspace4/1, Meas_Inv1/5  "<meas_i_out>"
  Bus Selector1/4 -> To Workspace3/1, Meas_Inv1/4  "<meas_i_inverter>"
  Bus Selector1/3 -> To Workspace2/1, Meas_Inv1/3  "<meas_u_out>"
  Bus Selector1/2 -> To Workspace1/1, Meas_Inv1/2  "<meas_u_cap>"
  Bus Selector1/1 -> To Workspace7/1, Meas_Inv1/1  "<meas_u_dc>"
  SimOut/1 -> Bus Selector1/1

== system VSM_specComp_DC_22a/VSM_4/VSM1/VSM ==
  cmd : Inport
  meas : Inport  Port=2
  BUS_GENERATION : Subsystem
  CONTROL : Subsystem
  MANAGEMENT : Subsystem  mask(VSMCC Management){Mgn=Ctrl.Mgn}
      mask prompts: Mgn "Mgn Parameters"
      mask help:
      | Mgn(.PQSpRateUp, .PQSpRateDown, PQSpMax, .PQSpMin)
      |
      | Parameter nicht auf der Maske:
      | ControlSampleTime
  Meas : Subsystem  mask(Messeinrichtung für VSM mit CC){PU=pu, PLL=Ctrl.PLL}
      mask prompts: PU "PU System"; PLL "PLL Parameters"
      mask help:
      | PU System(.Vb, .Ib)
      |
      | PLL Parameter (.kp, .ki)
      |
      | Parameter nicht auf der Maske:
      | NrChannels
      | ControlSampleTime
  ctrl : Outport  VectorParamsAs1DForOutWhenUnconnected=off  LockScale=on
  feedback : Outport  Port=2  VectorParamsAs1DForOutWhenUnconnected=off
  diag : Outport  Port=3  VectorParamsAs1DForOutWhenUnconnected=off
  wires:
  meas/1 -> Meas/1(MEASIN)
  cmd/1 -> MANAGEMENT/1(CMD)
  CONTROL/1(CONTROL) -> Meas/2("CONTROL "), BUS_GENERATION/2(CONTROL)
  BUS_GENERATION/1(ctrl) -> ctrl/1
  BUS_GENERATION/2(feedback) -> feedback/1
  CONTROL/2(diagCtrl) -> diag/1
  MANAGEMENT/1(MANAGE) -> CONTROL/1(MANAGE), BUS_GENERATION/1(MANAGE)
  Meas/1(MEAS) -> CONTROL/2(MEAS), MANAGEMENT/2(MEAS)

== system VSM_specComp_DC_22a/VSM_4/VSM1/command_center ==
  note: State Machine for TP <-> WP SIM
      |
      | State Index:
      | 0: Error
      | 1: Stop
      | 2: Ready (Precharge, Connected + Enable DC)
      | 3: Connect AC
      | 4: Enable AC
  Feed_AC : Inport
  Feed_DC : Inport  Port=2
  Bus Assignment : BusAssignment  AssignedSignals=Manage.connect,Manage.enable,Param.VSM.sp_PQ,Param.VSM.sp_E
  Bus Selector2 : BusSelector  OutputSignals=connect,enable
  Bus Creator1 : BusCreator  Inputs=2
  Constant2 : Constant  Value=1.01
  Display1 : Display
  Display2 : Display
  Display5 : Display
  Error ACK : Subsystem
      settings: OpenFcn=|
      | switch get_param([gcb '/Toggle'],'Value')
      |     case '1'
      |         set_param([gcb '/Toggle'],'Value', '0');
      |         set_param(gcb,'BackgroundColor','[0.8500    0.3250    0.0980]');
      |     case '0'
      |         set_param([gcb '/Toggle'],'Value', '1');
      |         set_param(gcb,'BackgroundColor','[0.4660    0.6740    0.1880]');
      | end
      mask Display: port_label('output',1,'')
  Rate Transition3 : RateTransition  Integrity=off  OutPortSampleTime=ControlSampleTime
  Shortcut1 : Subsystem  mask{path=./ControlLibrary/FriedrichLibrary.slx}
      settings: OpenFcn=findsimscopes
      mask Display: disp('Open Scopes...')
  Step3 : Step  Time=2  Before=[0.5 0]  After=[-0.5 0]  SampleTime=0
  Step4 : Step  Time=0  SampleTime=0
  Subsystem : Subsystem
  cmd_VSM : Subsystem  AncestorBlock=ControLibrary/cmd_VSM template
  cmd_tp : Outport  VectorParamsAs1DForOutWhenUnconnected=off
  cmd_ac : Outport  Port=2  VectorParamsAs1DForOutWhenUnconnected=off
  wires:
  Rate Transition3/1 -> cmd_ac/1
  cmd_VSM/1(cmd_ac) -> Bus Assignment/1
  Bus Assignment/1 -> Rate Transition3/1
  Error ACK/1(Out) -> Bus Creator1/1  "error_ack"
  Bus Creator1/1 -> cmd_tp/1
  Subsystem/1(precharge) -> Bus Creator1/2, Display5/1
  Feed_AC/1 -> Subsystem/1(In1)
  Feed_DC/1 -> Subsystem/2(In2)
  Subsystem/2(cmd_ac) -> Bus Selector2/1
  Step4/1 -> Subsystem/Enable
  Step3/1 -> Bus Assignment/4
  Constant2/1 -> Bus Assignment/5
  Bus Selector2/1 -> Display1/1, Bus Assignment/2  "<connect>"
  Bus Selector2/2 -> Display2/1, Bus Assignment/3  "<enable>"

== system VSM_specComp_DC_22a/VSM_4/VSM1/diagPlot ==
  Diag : Inport
  Add : Sum  Inputs=+-
  Bus Selector1 : BusSelector  OutputSignals=measDiag.PLL.f
  Bus Selector11 : BusSelector  OutputSignals=sp_i_dq,i_dq,enable_cc
  Bus Selector12 : BusSelector  OutputSignals=measDiag.PLL.vdq
  Bus Selector2 : BusSelector  OutputSignals=u_inv_dq,measDiag.u_cap.u_cap_dq0,measDiag.u_cap.u_cap_abc,manage.ENABLED
  Bus Selector3 : BusSelector  OutputSignals=u_inv_dq,measDiag.i_out.i_out_abc
  Bus Selector5 : BusSelector  OutputSignals=manage.sp_VSM.sp_PQ,measDiag.PQ,manage.sp_VSM.sp_f,vsmDiag.f
  Bus Selector6 : BusSelector  OutputSignals=vsmDiag.E
  Bus Selector7 : BusSelector  OutputSignals=pwmDiag.pwm,measDiag.i_inv.i_inv_abc,measDiag.PQ_out
  Bus Selector8 : BusSelector  OutputSignals=vsmDiag.sp_VSM.sp_E
  Bus Selector9 : BusSelector  OutputSignals=ccDiag
  Complex to Magnitude-Angle1 : ComplexToMagnitudeAngle  Commented=on
  Complex to Magnitude-Angle4 : ComplexToMagnitudeAngle
  Demux1 : Demux  Outputs=2
  Demux2 : Demux  Outputs=2
  Demux4 : Demux  Outputs=3
  Divide1 : Product  Inputs=/*
  Goto : Goto  Commented=on  GotoTag=Qref  TagVisibility=global
  Mux2 : Mux  Inputs=2
  Mux3 : Mux  Inputs=3
  Mux5 : Mux  Inputs=3
  Mux6 : Mux  Inputs=2
  PID Controller : slpidlib/PID Controller  Controller=PID  Form=Parallel  TimeDomain=Continuous-time  UseExternalTs=off  SampleTime=-1  IntegratorMethod=Forward Euler  FilterMethod=Forward Euler  ControllerParametersSource=internal  P=0.1  I=1  UseKiTs=off  D=0  N=100  UseFilter=on  TunerSelectOption=Transfer Function Based (PID Tuner App)  InitialConditionSource=internal  InitialConditionForIntegrator=1.085  InitialConditionForFilter=0  DifferentiatorICPrevScaledInput=0  ExternalReset=none  TrackingMode=off  Kt=1  LimitOutput=off  SatLimitsSource=internal  UpperSaturationLimit=inf  LowerSaturationLimit=-inf  LinearizeAsGain=on  AntiWindupMode=none  Kb=1  POutMin=[]  POutMax=[]  IOutMin=[]  IOutMax=[]  DOutMin=[]  DOutMax=[]  NOutMin=[]  NOutMax=[]  SumOutMin=[]  SumOutMax=[]  SaturationOutMin=[]  SaturationOutMax=[]  PParamMin=[]  PParamMax=[]  IParamMin=[]  IParamMax=[]  DParamMin=[]  DParamMax=[]  NParamMin=[]  NParamMax=[]  KbParamMin=[]  KbParamMax=[]  KtParamMin=[]  KtParamMax=[]  KbOutMin=[]  KbOutMax=[]  KtOutMin=[]  KtOutMax=[]  IntegratorOutMin=[]  IntegratorOutMax=[]  FilterOutMin=[]  FilterOutMax=[]  SumI1OutMin=[]  SumI1OutMax=[]  SumI2OutMin=[]  SumI2OutMax=[]  SumI3OutMin=[]  SumI3OutMax=[]  SumI4OutMin=[]  SumI4OutMax=[]  SumDOutMin=[]  SumDOutMax=[]  DifferentiatorOutMin=[]  DifferentiatorOutMax=[]  FilterDiffOutCoefMin=[]  FilterDiffOutCoefMax=[]  ReciprocalOutMin=[]  ReciprocalOutMax=[]  SumDenOutMin=[]  SumDenOutMax=[]  SumNumOutMin=[]  SumNumOutMax=[]  DivideOutMin=[]  DivideOutMax=[]  UdiffTsProdOutMin=[]  UdiffTsProdOutMax=[]  NTsProdOutMin=[]  NTsProdOutMax=[]  UintegralTsProdOutMin=[]  UintegralTsProdOutMax=[]  UngainTsProdOutMin=[]  UngainTsProdOutMax=[]  IntegratorContinuousStateAttributes=''  IntegratorStateMustResolveToSignalObject=off  IntegratorRTWStateStorageClass=Auto  FilterContinuousStateAttributes=''  FilterStateMustResolveToSignalObject=off  FilterRTWStateStorageClass=Auto  ParallelPVariant=InternalParameters  IdealPVariant=Disabled  IVariant=InternalParameters  DVariant=InternalParameters  IntegratorVariant=Continuous  SatVariant=Disabled  AWVariant=Passthrough  PCopyVariant=Disabled  TRVariant=Disabled  FdbkBlocksVariant=Forward  IdealPFdbkVariant=Disabled  SatFdbkVariant=Disabled  DerivativeFilterVariant=ContFilter  NVariant=InternalParameters  NCopyVariant=Disabled  FilterICVariant=InternalICsFilter  IntegratorICVariant=InternalICs  ExternalResetVariant=Disabled  TRSumVariant=Passthrough  SumFdbkVariant=Disabled  SumVariant=Sum_PID  TsampFilterVariant=InternalTs  TsampNgainVariant=Passthrough  TsampIntegralVariant=Disabled_SignalSpec  ExternalSaturationOutDataTypeStr=Inherit: Same as second input
  Product : Product
  Product1 : Product
  Real-Imag to Complex1 : RealImagToComplex  Commented=on
  Real-Imag to Complex4 : RealImagToComplex
  Scope : Scope  Commented=on  NumInputPorts=2
  Scope1 : Scope  NumInputPorts=2
  Scope6 : Scope  NumInputPorts=4
  Signal Specification{1,5..10} (7 alike) : SignalSpecification
  Step : Step  Time=6+10  Before=0.1  After=0.5  SampleTime=0
  Step1 : Step  Time=6+10  SampleTime=0
  VSM ctrl PQ f : Scope  NumInputPorts=3
  VSM ctrl PQ f1 : Scope  Commented=on  NumInputPorts=4
  VSM_pwm : Scope  Commented=on  NumInputPorts=3
  "[40 60] Hz" : Saturate  UpperLimit=60  LowerLimit=40
  cc_ctrl : Scope  NumInputPorts=3
  dq->abs1 : Subsystem
  dq0 : Scope  Commented=on  NumInputPorts=4
  dq0->abs : Subsystem
  dq0->abs2 : Subsystem
  rPQ : Scope  Commented=on  NumInputPorts=2
  wires:
  Diag/1 -> Bus Selector2/1, Bus Selector6/1, Bus Selector7/1, Bus Selector3/1, Bus Selector9/1, Bus Selector12/1, Bus Selector8/1, Bus Selector1/1, Bus Selector5/1
  Bus Selector7/1 -> VSM_pwm/1  "<pwm>"
  Mux5/1 -> VSM ctrl PQ f/3
  dq0->abs/1(abs) -> Mux5/2  "abs_vc"
  Bus Selector8/1 -> Signal Specification10/1  "<sp_E>"
  Bus Selector11/1 -> Mux6/1  "<sp_i_dq>"
  Bus Selector9/1 -> Bus Selector11/1  "<ccDiag>"
  Bus Selector12/1 -> dq0->abs/1(dq0)  "<vdq>"
  Bus Selector11/3 -> VSM ctrl PQ f1/4, cc_ctrl/3  "<enable_cc>"
  Mux6/1 -> Scope6/2, cc_ctrl/1
  Bus Selector5/1 -> Signal Specification5/1  "<sp_PQ>"
  Bus Selector5/2 -> Signal Specification6/1  "<PQ>"
  Bus Selector5/3 -> Signal Specification7/1  "<sp_f>"
  Bus Selector5/4 -> Signal Specification8/1  "<f>"
  Signal Specification5/1 -> Mux2/1  "PQ_sp"
  Signal Specification7/1 -> Mux3/1  "f_sp"
  Signal Specification8/1 -> VSM ctrl PQ f1/3, Mux3/2  "f_vsm"
  Mux2/1 -> VSM ctrl PQ f/1
  Mux3/1 -> "[40 60] Hz"/1
  Bus Selector1/1 -> Signal Specification9/1  "<f>"
  Signal Specification9/1 -> Mux3/3  "f_pll"
  Signal Specification10/1 -> Mux5/1  "vsm_E_sp"
  Bus Selector11/2 -> dq->abs1/1(dq), Mux6/2  "<i_dq>"
  dq->abs1/1(abs) -> cc_ctrl/2, Scope6/4
  Bus Selector6/1 -> Signal Specification1/1  "<E>"
  Signal Specification1/1 -> Mux5/3  "vsm_E"
  "[40 60] Hz"/1 -> VSM ctrl PQ f/2
  dq0->abs2/1(abs) -> Scope6/1, dq0/4  "|u|"
  Bus Selector3/2 -> VSM_pwm/3, rPQ/2  "<i_out_abc>"
  Bus Selector3/1 -> rPQ/1  "<u_inv_dq>"
  Bus Selector7/2 -> VSM_pwm/2  "<i_inv_abc>"
  Bus Selector2/2 -> dq0->abs2/1(dq0), Demux4/1, dq0/2  "<u_cap_dq0>"
  Real-Imag to Complex4/1 -> Complex to Magnitude-Angle4/1
  Demux4/1 -> Real-Imag to Complex4/1
  Demux4/2 -> Real-Imag to Complex4/2
  Complex to Magnitude-Angle4/1 -> Divide1/1  "cap"
  Signal Specification6/1 -> Demux2/1, VSM ctrl PQ f1/2, Mux2/2  "PQ"
  Bus Selector7/3 -> Divide1/2  "<PQ_out>"
  Divide1/1 -> Scope/1, Scope6/3
  Demux1/2 -> Real-Imag to Complex1/2
  Demux1/1 -> Real-Imag to Complex1/1
  Real-Imag to Complex1/1 -> Complex to Magnitude-Angle1/1
  Complex to Magnitude-Angle1/2 -> Scope/2  "U_cap"
  Bus Selector2/1 -> Demux1/1, dq0/3, dq0/1  "<u_inv_dq>"
  Demux2/2 -> Add/2
  PID Controller/1 -> Scope1/1, Goto/1
  Step/1 -> Product/2
  Product/1 -> Add/1
  Bus Selector2/4 -> Scope1/2, Product/1  "<ENABLED>"
  Add/1 -> Product1/2
  Product1/1 -> PID Controller/1
  Step1/1 -> Product1/1

== system VSM_specComp_DC_22a/VSM_1/VSM1/VSM/BUS_GENERATION ==
  MANAGE : Inport
  CONTROL : Inport  Port=2
  Bus Creator1 : BusCreator  Inputs=4
  Bus Selector2 : BusSelector  OutputSignals=PWM
  Bus Selector3 : BusSelector  OutputSignals=ENABLED,CONNECT
  Bus Selector4 : BusSelector  OutputSignals=CONNECTED,ENABLED
  Bus Creator6 : BusCreator  Inputs=2  OutDataTypeStr=Bus: FeedbackACBus
  Data Type Conversion{,1..3} (4 alike) : DataTypeConversion  SaturateOnIntegerOverflow=off  RndMeth=Floor
  Signal Specification1 : SignalSpecification
  additional data1 : Constant  Value=0
  ctrl : Outport  VectorParamsAs1DForOutWhenUnconnected=off
  feedback : Outport  Port=2  VectorParamsAs1DForOutWhenUnconnected=off
  wires:
  Data Type Conversion3/1 -> Bus Creator6/1  "connected"
  Bus Selector3/2 -> Data Type Conversion1/1  "<CONNECT>"
  additional data1/1 -> Bus Creator1/4  "source_id"
  Data Type Conversion1/1 -> Bus Creator1/3  "connect"
  Data Type Conversion/1 -> Bus Creator1/2  "enable"
  Bus Selector3/1 -> Data Type Conversion/1  "<ENABLED>"
  Bus Creator6/1 -> feedback/1
  Bus Creator1/1 -> ctrl/1
  MANAGE/1 -> Bus Selector4/1, Bus Selector3/1
  Signal Specification1/1 -> Bus Creator1/1  "pwm"
  Data Type Conversion2/1 -> Bus Creator6/2  "enabled"
  CONTROL/1 -> Bus Selector2/1
  Bus Selector4/2 -> Data Type Conversion2/1  "<ENABLED>"
  Bus Selector4/1 -> Data Type Conversion3/1  "<CONNECTED>"
  Bus Selector2/1 -> Signal Specification1/1  "<PWM>"
